simulink model "FuzzyModel"  (Simulink 8.5)
settings: Solver=ode45  StartTime=0.0  StopTime=10.0  RelTol=1e-3
libraries: fuzblock x1
settings Model: Creator=YH  LastModifiedBy=YH
settings DataIOCC: SignalLoggingSaveFormat=Dataset
settings OptimizationCC: ExpressionDepthLimit=128
settings DebuggingCC: UnderspecifiedInitializationDetection=Simplified  MergeDetectMultiDrivingBlocksExec=error  FcnCallInpInsideContextMsg=EnableAllAsError  StateNameClashWarn=none
settings GRTTargetCC: CombineOutputUpdateFcns=on  GRTInterface=off

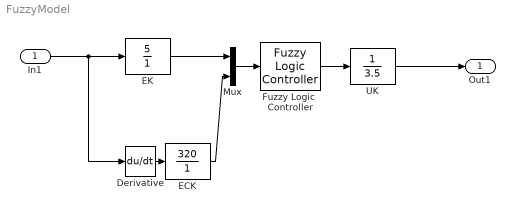
== system FuzzyModel ==
  In1 : Inport
  Derivative : Derivative
  "ECK " : TransferFcn  Numerator=[320]  Denominator=[1]
  EK : TransferFcn  Numerator=[5]  Denominator=[1]
  Fuzzy Logic  Controller : fuzblock/Fuzzy Logic  Controller  RequirementInfo={} %GIDa_313f7fb3_81d9_41ef_bb04_96940627a228  fis=fuzzyController
  Mux : Mux  Inputs=2
  UK : TransferFcn  Denominator=[3.5]
  Out1 : Outport
  wires:
  Derivative/1 -> "ECK "/1
  Mux/1 -> Fuzzy Logic  Controller/1
  Fuzzy Logic  Controller/1 -> UK/1
  EK/1 -> Mux/1
  "ECK "/1 -> Mux/2
  In1/1 -> Derivative/1, EK/1
  UK/1 -> Out1/1
